simulink model "PMSM_FOC_Model"  (R2021a)
settings: Solver=FixedStepDiscrete  StartTime=0.0  StopTime=4  FixedStep=0.0001  RelTol=1e-3
settings Model: Creator=Wu  LastModifiedBy=Wu

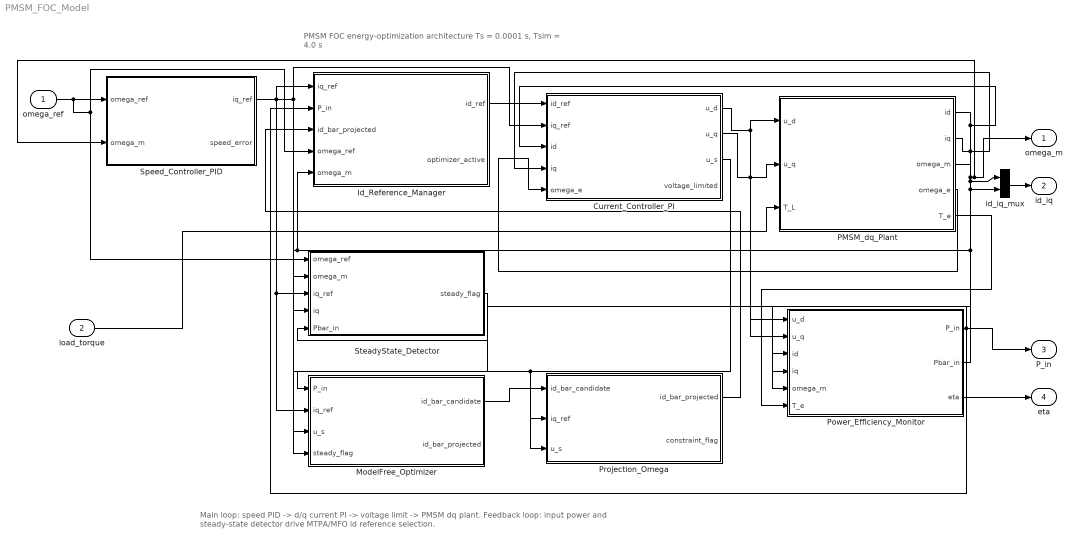
== system PMSM_FOC_Model ==
  note: PMSM FOC energy-optimization architecture
      | Ts = 0.0001 s, Tsim = 4.0 s
  note: Main loop: speed PID -> d/q current PI -> voltage limit -> PMSM dq plant. Feedback loop: input power and steady-state detector drive MTPA/MFO id reference selection.
  omega_ref : Inport
  load_torque : Inport  Port=2
  Current_Controller_PI : Subsystem
  Id_Reference_Manager : Subsystem
  ModelFree_Optimizer : Subsystem
  PMSM_dq_Plant : Subsystem
  Power_Efficiency_Monitor : Subsystem
  Projection_Omega : Subsystem
  Speed_Controller_PID : Subsystem
  SteadyState_Detector : Subsystem
  id_iq_mux : Mux  Inputs=2
  omega_m : Outport
  id_iq : Outport  Port=2
  P_in : Outport  Port=3
  eta : Outport  Port=4
  wires:
  omega_ref/1 -> Id_Reference_Manager/4(omega_ref), SteadyState_Detector/1(omega_ref), Speed_Controller_PID/1(omega_ref)
  Speed_Controller_PID/1(iq_ref) -> SteadyState_Detector/3(iq_ref), ModelFree_Optimizer/2(iq_ref), Current_Controller_PI/2(iq_ref), Projection_Omega/2(iq_ref), Id_Reference_Manager/1(iq_ref)
  Id_Reference_Manager/1(id_ref) -> Current_Controller_PI/1(id_ref)
  Current_Controller_PI/1(u_d) -> Power_Efficiency_Monitor/1(u_d), PMSM_dq_Plant/1(u_d)
  Current_Controller_PI/2(u_q) -> Power_Efficiency_Monitor/2(u_q), PMSM_dq_Plant/2(u_q)
  load_torque/1 -> PMSM_dq_Plant/3(T_L)
  PMSM_dq_Plant/1(id) -> Power_Efficiency_Monitor/3(id), id_iq_mux/1, Current_Controller_PI/3(id)
  PMSM_dq_Plant/2(iq) -> Power_Efficiency_Monitor/4(iq), SteadyState_Detector/4(iq), id_iq_mux/2, Current_Controller_PI/4(iq)
  PMSM_dq_Plant/3(omega_m) -> Id_Reference_Manager/5(omega_m), SteadyState_Detector/2(omega_m), Power_Efficiency_Monitor/5(omega_m), Speed_Controller_PID/2(omega_m), omega_m/1
  PMSM_dq_Plant/4(omega_e) -> Current_Controller_PI/5(omega_e)
  PMSM_dq_Plant/5(T_e) -> Power_Efficiency_Monitor/6(T_e)
  Power_Efficiency_Monitor/2(Pbar_in) -> SteadyState_Detector/5(Pbar_in)
  Power_Efficiency_Monitor/1(P_in) -> ModelFree_Optimizer/1(P_in), Id_Reference_Manager/2(P_in), P_in/1
  Current_Controller_PI/3(u_s) -> ModelFree_Optimizer/3(u_s), Projection_Omega/3(u_s)
  SteadyState_Detector/1(steady_flag) -> ModelFree_Optimizer/4(steady_flag)
  ModelFree_Optimizer/1(id_bar_candidate) -> Projection_Omega/1(id_bar_candidate)
  Projection_Omega/1(id_bar_projected) -> Id_Reference_Manager/3(id_bar_projected)
  id_iq_mux/1 -> id_iq/1
  Power_Efficiency_Monitor/3(eta) -> eta/1

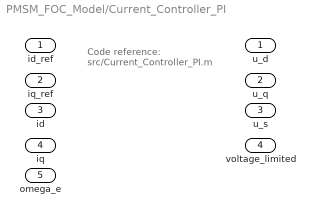
== system PMSM_FOC_Model/Current_Controller_PI ==
  note: Code reference:
      | src/Current_Controller_PI.m
  id_ref : Inport
  iq_ref : Inport  Port=2
  id : Inport  Port=3
  iq : Inport  Port=4
  omega_e : Inport  Port=5
  u_d : Outport
  u_q : Outport  Port=2
  u_s : Outport  Port=3
  voltage_limited : Outport  Port=4

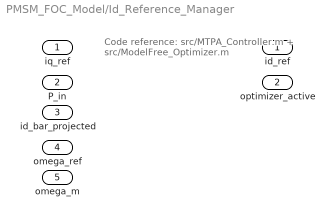
== system PMSM_FOC_Model/Id_Reference_Manager ==
  note: Code reference:
      | src/MTPA_Controller.m + src/ModelFree_Optimizer.m
  iq_ref : Inport
  P_in : Inport  Port=2
  id_bar_projected : Inport  Port=3
  omega_ref : Inport  Port=4
  omega_m : Inport  Port=5
  id_ref : Outport
  optimizer_active : Outport  Port=2

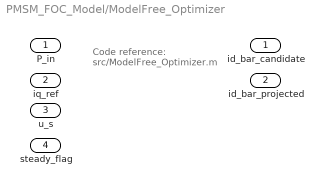
== system PMSM_FOC_Model/ModelFree_Optimizer ==
  note: Code reference:
      | src/ModelFree_Optimizer.m
  P_in : Inport
  iq_ref : Inport  Port=2
  u_s : Inport  Port=3
  steady_flag : Inport  Port=4
  id_bar_candidate : Outport
  id_bar_projected : Outport  Port=2

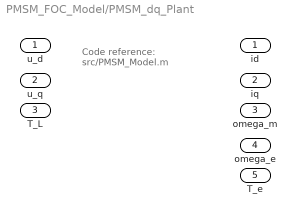
== system PMSM_FOC_Model/PMSM_dq_Plant ==
  note: Code reference:
      | src/PMSM_Model.m
  u_d : Inport
  u_q : Inport  Port=2
  T_L : Inport  Port=3
  id : Outport
  iq : Outport  Port=2
  omega_m : Outport  Port=3
  omega_e : Outport  Port=4
  T_e : Outport  Port=5

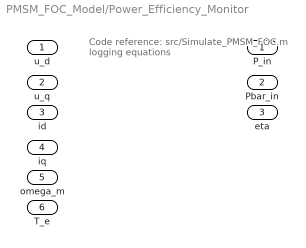
== system PMSM_FOC_Model/Power_Efficiency_Monitor ==
  note: Code reference:
      | src/Simulate_PMSM_FOC.m logging equations
  u_d : Inport
  u_q : Inport  Port=2
  id : Inport  Port=3
  iq : Inport  Port=4
  omega_m : Inport  Port=5
  T_e : Inport  Port=6
  P_in : Outport
  Pbar_in : Outport  Port=2
  eta : Outport  Port=3

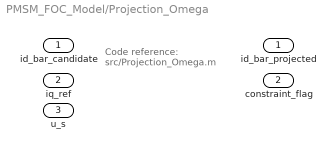
== system PMSM_FOC_Model/Projection_Omega ==
  note: Code reference:
      | src/Projection_Omega.m
  id_bar_candidate : Inport
  iq_ref : Inport  Port=2
  u_s : Inport  Port=3
  id_bar_projected : Outport
  constraint_flag : Outport  Port=2

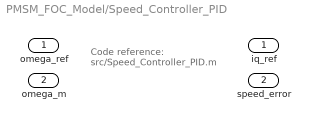
== system PMSM_FOC_Model/Speed_Controller_PID ==
  note: Code reference:
      | src/Speed_Controller_PID.m
  omega_ref : Inport
  omega_m : Inport  Port=2
  iq_ref : Outport
  speed_error : Outport  Port=2

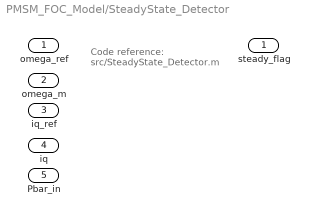
== system PMSM_FOC_Model/SteadyState_Detector ==
  note: Code reference:
      | src/SteadyState_Detector.m
  omega_ref : Inport
  omega_m : Inport  Port=2
  iq_ref : Inport  Port=3
  iq : Inport  Port=4
  Pbar_in : Inport  Port=5
  steady_flag : Outport
